simulink model "LAB1_Model1DOF_Controller"  (R2021a)
settings: Solver=VariableStepAuto  StartTime=0.0  StopTime=5  RelTol=1e-3
libraries: fl_lib x9, nesl_utility x6, dspfdesign x2, pid_lib x2, ee_lib x1, simulink x1
settings Model: Creator=matas  LastModifiedBy=10907
settings SolverCC: AlgebraicLoopSolver=TrustRegion
settings DebuggingCC: SFMachineParentedDataDiag=warning

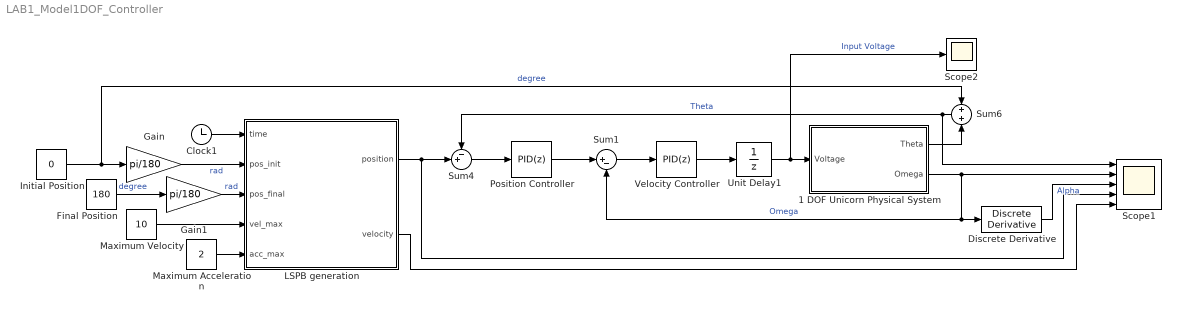
== system LAB1_Model1DOF_Controller ==
  1 DOF Unicorn Physical System : Subsystem  mask{I=0.1, b=0.01}
      mask prompts: I "Inertia"; b "Damping"
  Clock1 : Clock
  Discrete Derivative : simulink/Discrete/Discrete Derivative  gainval=1.0  ICPrevScaledInput=0.0  OutMin=[]  OutMax=[]  OutDataType=fixdt(1, 16)  OutScaling=2^-10  DoSatur=off
  Final Position : Constant  Value=180
  Gain : Gain  Gain=pi/180
  Gain1 : Gain  Gain=pi/180
  Initial Position : Constant  Value=0
  LSPB generation : MATLAB Function  TreatAsAtomicUnit=on
  Maximum Acceleration : Constant  Value=2
  Maximum Velocity : Constant  Value=10
  Position Controller : pid_lib/PID Controller  Controller=PID  Form=Parallel  TimeDomain=Discrete-time  UseExternalTs=off  SampleTime=1e-3  IntegratorMethod=Forward Euler  FilterMethod=Forward Euler  ControllerParametersSource=internal  P=150  I=100  D=10  UseFilter=on  N=100  TunerSelectOption=Transfer Function Based (PID Tuner App)  InitialConditionSource=internal  InitialConditionForIntegrator=0  InitialConditionForFilter=0  DifferentiatorICPrevScaledInput=0  ExternalReset=none  TrackingMode=off  Kt=1  LimitOutput=off  SatLimitsSource=internal  UpperSaturationLimit=2  LowerSaturationLimit=0  LinearizeAsGain=off  AntiWindupMode=none  Kb=1  POutMin=[]  POutMax=[]  IOutMin=[]  IOutMax=[]  DOutMin=[]  DOutMax=[]  NOutMin=[]  NOutMax=[]  SumOutMin=[]  SumOutMax=[]  SaturationOutMin=[]  SaturationOutMax=[]  PParamMin=[]  PParamMax=[]  IParamMin=[]  IParamMax=[]  DParamMin=[]  DParamMax=[]  NParamMin=[]  NParamMax=[]  KbParamMin=[]  KbParamMax=[]  KtParamMin=[]  KtParamMax=[]  KbOutMin=[]  KbOutMax=[]  KtOutMin=[]  KtOutMax=[]  IntegratorOutMin=[]  IntegratorOutMax=[]  FilterOutMin=[]  FilterOutMax=[]  SumI1OutMin=[]  SumI1OutMax=[]  SumI2OutMin=[]  SumI2OutMax=[]  SumI3OutMin=[]  SumI3OutMax=[]  SumI4OutMin=[]  SumI4OutMax=[]  SumDOutMin=[]  SumDOutMax=[]  DifferentiatorOutMin=[]  DifferentiatorOutMax=[]  FilterDiffOutCoefMin=[]  FilterDiffOutCoefMax=[]  ReciprocalOutMin=[]  ReciprocalOutMax=[]  SumDenOutMin=[]  SumDenOutMax=[]  SumNumOutMin=[]  SumNumOutMax=[]  DivideOutMin=[]  DivideOutMax=[]  UdiffTsProdOutMin=[]  UdiffTsProdOutMax=[]  NTsProdOutMin=[]  NTsProdOutMax=[]  UintegralTsProdOutMin=[]  UintegralTsProdOutMax=[]  UngainTsProdOutMin=[]  UngainTsProdOutMax=[]  IntegratorContinuousStateAttributes=''  IntegratorStateMustResolveToSignalObject=off  IntegratorRTWStateStorageClass=Auto  FilterContinuousStateAttributes=''  FilterStateMustResolveToSignalObject=off  FilterRTWStateStorageClass=Auto  ParallelPVariant=InternalParameters  IdealPVariant=Disabled  IVariant=InternalParameters  DVariant=InternalParameters  IntegratorVariant=Discrete  SatVariant=Disabled  AWVariant=Passthrough  PCopyVariant=Disabled  TRVariant=Disabled  FdbkBlocksVariant=Forward  IdealPFdbkVariant=Disabled  SatFdbkVariant=Disabled  DerivativeFilterVariant=ForwardEulerFilter  NVariant=InternalParameters  NCopyVariant=Disabled  FilterICVariant=InternalICsFilter  IntegratorICVariant=InternalICs  ExternalResetVariant=Disabled  TRSumVariant=Passthrough  SumFdbkVariant=Disabled  SumVariant=Sum_PID  TsampFilterVariant=InternalTs  TsampNgainVariant=Passthrough  TsampIntegralVariant=Passthrough  ExternalSaturationOutDataTypeStr=Inherit: Same as second input
  Scope1 : Scope  NumInputPorts=5
  Scope2 : Scope
  Sum1 : Sum  Inputs=|+-
  Sum4 : Sum  Inputs=-+|
  Sum6 : Sum  Inputs=+|+
  Unit Delay1 : UnitDelay  SampleTime=1/1000  HasFrameUpgradeWarning=on
  Velocity Controller : pid_lib/PID Controller  Controller=PID  Form=Parallel  TimeDomain=Discrete-time  UseExternalTs=off  SampleTime=1e-3  IntegratorMethod=Forward Euler  FilterMethod=Forward Euler  ControllerParametersSource=internal  P=0.05  I=0.5  D=0  UseFilter=on  N=100  TunerSelectOption=Transfer Function Based (PID Tuner App)  InitialConditionSource=internal  InitialConditionForIntegrator=0  InitialConditionForFilter=0  DifferentiatorICPrevScaledInput=0  ExternalReset=none  TrackingMode=off  Kt=1  LimitOutput=off  SatLimitsSource=internal  UpperSaturationLimit=2  LowerSaturationLimit=0  LinearizeAsGain=off  AntiWindupMode=none  Kb=1  POutMin=[]  POutMax=[]  IOutMin=[]  IOutMax=[]  DOutMin=[]  DOutMax=[]  NOutMin=[]  NOutMax=[]  SumOutMin=[]  SumOutMax=[]  SaturationOutMin=[]  SaturationOutMax=[]  PParamMin=[]  PParamMax=[]  IParamMin=[]  IParamMax=[]  DParamMin=[]  DParamMax=[]  NParamMin=[]  NParamMax=[]  KbParamMin=[]  KbParamMax=[]  KtParamMin=[]  KtParamMax=[]  KbOutMin=[]  KbOutMax=[]  KtOutMin=[]  KtOutMax=[]  IntegratorOutMin=[]  IntegratorOutMax=[]  FilterOutMin=[]  FilterOutMax=[]  SumI1OutMin=[]  SumI1OutMax=[]  SumI2OutMin=[]  SumI2OutMax=[]  SumI3OutMin=[]  SumI3OutMax=[]  SumI4OutMin=[]  SumI4OutMax=[]  SumDOutMin=[]  SumDOutMax=[]  DifferentiatorOutMin=[]  DifferentiatorOutMax=[]  FilterDiffOutCoefMin=[]  FilterDiffOutCoefMax=[]  ReciprocalOutMin=[]  ReciprocalOutMax=[]  SumDenOutMin=[]  SumDenOutMax=[]  SumNumOutMin=[]  SumNumOutMax=[]  DivideOutMin=[]  DivideOutMax=[]  UdiffTsProdOutMin=[]  UdiffTsProdOutMax=[]  NTsProdOutMin=[]  NTsProdOutMax=[]  UintegralTsProdOutMin=[]  UintegralTsProdOutMax=[]  UngainTsProdOutMin=[]  UngainTsProdOutMax=[]  IntegratorContinuousStateAttributes=''  IntegratorStateMustResolveToSignalObject=off  IntegratorRTWStateStorageClass=Auto  FilterContinuousStateAttributes=''  FilterStateMustResolveToSignalObject=off  FilterRTWStateStorageClass=Auto  ParallelPVariant=InternalParameters  IdealPVariant=Disabled  IVariant=InternalParameters  DVariant=InternalParameters  IntegratorVariant=Discrete  SatVariant=Disabled  AWVariant=Passthrough  PCopyVariant=Disabled  TRVariant=Disabled  FdbkBlocksVariant=Forward  IdealPFdbkVariant=Disabled  SatFdbkVariant=Disabled  DerivativeFilterVariant=ForwardEulerFilter  NVariant=InternalParameters  NCopyVariant=Disabled  FilterICVariant=InternalICsFilter  IntegratorICVariant=InternalICs  ExternalResetVariant=Disabled  TRSumVariant=Passthrough  SumFdbkVariant=Disabled  SumVariant=Sum_PID  TsampFilterVariant=InternalTs  TsampNgainVariant=Passthrough  TsampIntegralVariant=Passthrough  ExternalSaturationOutDataTypeStr=Inherit: Same as second input
  wires:
  Final Position/1 -> Gain1/1  "degree"
  Initial Position/1 -> Sum6/1, Gain/1  "degree"
  Maximum Acceleration/1 -> LSPB generation/5(acc_max)
  Maximum Velocity/1 -> LSPB generation/4(vel_max)
  Clock1/1 -> LSPB generation/1(time)
  LSPB generation/2(velocity) -> Scope1/5
  LSPB generation/1(position) -> Sum4/2, Scope1/4
  Velocity Controller/1 -> Unit Delay1/1
  1 DOF Unicorn Physical System/2(Omega) -> Discrete Derivative/1, Sum1/2, Scope1/2  "Omega"
  1 DOF Unicorn Physical System/1(Theta) -> Sum6/2
  Sum1/1 -> Velocity Controller/1
  Sum4/1 -> Position Controller/1
  Position Controller/1 -> Sum1/1
  Unit Delay1/1 -> Scope2/1, 1 DOF Unicorn Physical System/1(Voltage)  "Input Voltage"
  Discrete Derivative/1 -> Scope1/3  "Alpha"
  Sum6/1 -> Scope1/1, Sum4/1  "Theta"
  Gain/1 -> LSPB generation/2(pos_init)  "rad"
  Gain1/1 -> LSPB generation/3(pos_final)  "rad"

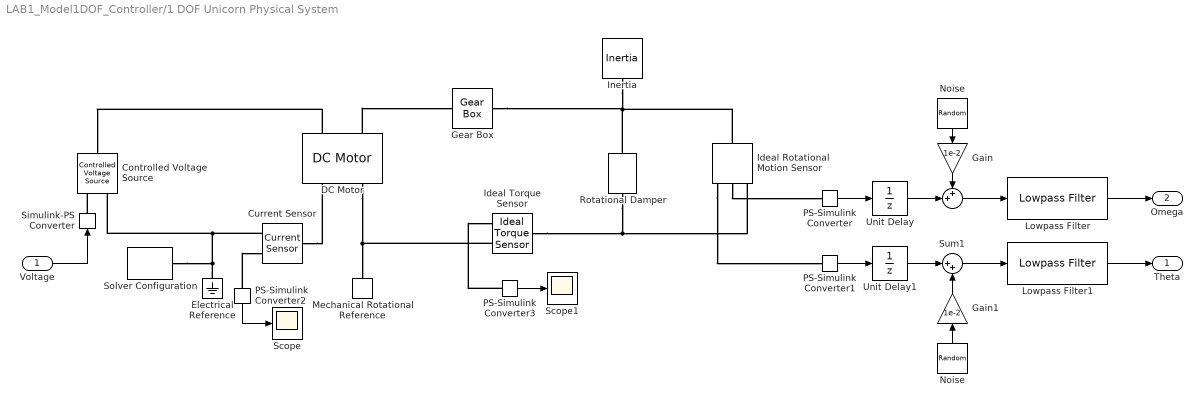
== system LAB1_Model1DOF_Controller/1 DOF Unicorn Physical System ==
  Voltage : Inport
  " " : Sum  Inputs=++|
  Controlled Voltage Source : fl_lib/Electrical/Electrical Sources/Controlled Voltage Source
  Current Sensor : fl_lib/Electrical/Electrical Sensors/Current Sensor
  "DC Motor " : ee_lib/Electromechanical/Brushed Motors/DC Motor  field_option=ee.enum.field_option.pm  Rf=100 Ohm  Lf=1 H  Laf=0.15 H  If0=0 A  parameterization=ee.enum.dcparam_option.load_speed  Ra=3.9 Ohm  La=65 uH  emf_or_torque=ee.enum.emf_or_torque.kv  Kv=0.072e-3 V/rpm  Ki=6.876e-4 N*m/A  T_stall=0.24e-3 N*m  w_max=8100 rpm  w_rated=7700 rpm  P_rated=17 W  V_rated=12 V  J=0.01 g*cm^2  lam_param=ee.enum.lam_param.current  lam=0 N*m/(rad/s)  i_noload=0.075 A  V_i_noload=12 V  speed0=0 rpm  enable_fault_armature=ee.enum.faults.faultEnable.no  rev_faulted=1 / 3  G_faulted_armature=1e-5 S  fault_trigger_armature=ee.enum.faults.faultTrigger.temporal  t_fault_armature=1 s  max_permissible_current_armature=inf A  t_fail_on_current_armature=1 s  enable_fault_field=ee.enum.faults.faultEnable.no  G_faulted_field=1e-5 S  fault_trigger_field=ee.enum.faults.faultTrigger.temporal  t_fault_field=1 s  max_permissible_current_field=inf A  t_fail_on_current_field=1 s  fault_action=ee.enum.faults.faultAction.none  alpha=3.93e-3 1/K  Tmeas=25 degC  thermal_mass=100 J/K  initial_temperature=25 degC
  Electrical Reference : fl_lib/Electrical/Electrical Elements/Electrical Reference
  Gain : Gain  Gain=1e-2
  Gain1 : Gain  Gain=1e-2
  Gear Box : fl_lib/Mechanical/Mechanisms/Gear Box  ratio=64  t_in_specify=off  t_in_priority=None  t_in=0 N*m  t_in_nominal_specify=off  t_in_nominal_unit=N*m  t_in_nominal_value=1  t_out_specify=off  t_out_priority=None  t_out=0 N*m  t_out_nominal_specify=off  t_out_nominal_unit=N*m  t_out_nominal_value=1
  Ideal Rotational Motion Sensor : fl_lib/Mechanical/Mechanical Sensors/Ideal Rotational Motion Sensor  wrap_angle=simscape.enum.onoff.off  offset=0 rad
  Ideal Torque Sensor : fl_lib/Mechanical/Mechanical Sensors/Ideal Torque Sensor
  Inertia : fl_lib/Mechanical/Rotational Elements/Inertia  inertia=I kg*m^2  num_ports=foundation.enum.numPorts2.one  w_specify=off  w_priority=High  w=0 rad/s  w_nominal_specify=off  w_nominal_unit=rad/s  w_nominal_value=1  t_specify=off  t_priority=None  t=0 N*m  t_nominal_specify=off  t_nominal_unit=N*m  t_nominal_value=1
  Lowpass Filter : dspfdesign/Lowpass Filter  FilterType=FIR  DesignForMinimumOrder=on  FilterOrder=50  PassbandFrequency=1.6  StopbandFrequency=30  PassbandRipple=0.1  StopbandAttenuation=40  InheritSampleRate=on  SampleRate=44100  SimulateUsing=Interpreted execution  roundingMode=Floor  coeffsDataTypeStr=fixdt(1,16)
  Lowpass Filter1 : dspfdesign/Lowpass Filter  FilterType=FIR  DesignForMinimumOrder=on  FilterOrder=50  PassbandFrequency=1.6  StopbandFrequency=30  PassbandRipple=0.1  StopbandAttenuation=40  InheritSampleRate=on  SampleRate=44100  SimulateUsing=Interpreted execution  roundingMode=Floor  coeffsDataTypeStr=fixdt(1,16)
  Mechanical Rotational Reference : fl_lib/Mechanical/Rotational Elements/Mechanical Rotational Reference
  Noise : RandomNumber  Variance=1/100000  SampleTime=1/1000
  "Noise " : RandomNumber  Variance=1/100000  SampleTime=1/100
  PS-Simulink Converter{,1..3} (4 alike) : nesl_utility/PS-Simulink Converter  PhysicalDomain=network_engine_domain  SubClassName=ps_output  LeftPortType=input  RightPortType=output  PseudoPeriodic=off  Frequencies=[]  Unit=inherit  AffineConversion=off
      settings: SourceProductBaseCode=PW,SS
  Rotational Damper : fl_lib/Mechanical/Rotational Elements/Rotational Damper  D=b N*m/(rad/s)  w_specify=off  w_priority=None  w=0 rad/s  w_nominal_specify=off  w_nominal_unit=rad/s  w_nominal_value=1  t_specify=off  t_priority=None  t=0 N*m  t_nominal_specify=off  t_nominal_unit=N*m  t_nominal_value=1
  Scope : Scope
  Scope1 : Scope
  Simulink-PS Converter : nesl_utility/Simulink-PS Converter  PhysicalDomain=network_engine_domain  SubClassName=ps_input  LeftPortType=input  RightPortType=output  PseudoPeriodic=off  Frequencies=[]  NoiseDistribution=none  NoiseParameters=[]  Unit=1  AffineConversion=off  FilteringAndDerivatives=provide  SimscapeFilterOrder=1  InputFilterTimeConstant=0.001  UdotUserProvided=0
      settings: SourceProductBaseCode=PW,SS
  Solver Configuration : nesl_utility/Solver Configuration  PhysicalDomain=network_engine_domain  SubClassName=solver  LeftPortType=input  RightPortType=generic  Tones=[]  Harmonics=[]  SimulateNoise=off  Profile=off  UseLocalSampling=off  EnableSwitchedLinearOptims=on  FrequencyDomain=off  UseCCode=off  RelTol=0.001  AbsTol=1e-06  MinStep=1e-09  ToWorkspace=off  RevertToSquareIcSolve=off  NumHomotopyIterations=100  PhasorMode=off  PhasorModeNumHarmonics=1  DoDC=off  ResidualTolerance=1e-09  UseLocalSolver=off  LocalSolverChoice=NE_BACKWARD_EULER_ADVANCER  LocalSolverSampleTime=0.001  DoFixedCost=off  MaxNonlinIter=3  MaxModeIter=2  ComputeImpulses=off  ImpulseIterations=2  LinearAlgebra=auto  EquationFormulation=NE_TIME_EF  DelaysMemoryBudget=1024  AutomaticFiltering=on  FilteringTimeConstant=0.001  PartitionStorageMethod=AS_NEEDED  PartitionMemoryBudget=1024  PartitionMethod=ROBUST
      settings: SourceProductBaseCode=PW,SS
  Sum1 : Sum  Inputs=|++
  Unit Delay : UnitDelay  SampleTime=1/1000  HasFrameUpgradeWarning=on
  Unit Delay1 : UnitDelay  SampleTime=1/1000  HasFrameUpgradeWarning=on
  Theta : Outport
  Omega : Outport  Port=2
  wires:
  PS-Simulink Converter/1 -> Unit Delay/1
  PS-Simulink Converter2/1 -> Scope/1
  PS-Simulink Converter3/1 -> Scope1/1
  Noise/1 -> Gain/1
  Unit Delay/1 -> " "/2
  Lowpass Filter/1 -> Omega/1
  "Noise "/1 -> Gain1/1
  Unit Delay1/1 -> Sum1/1
  Sum1/1 -> Lowpass Filter1/1
  PS-Simulink Converter1/1 -> Unit Delay1/1
  Lowpass Filter1/1 -> Theta/1
  Voltage/1 -> Simulink-PS Converter/1
  " "/1 -> Lowpass Filter/1
  Gain1/1 -> Sum1/2
  Gain/1 -> " "/1
  connections:
  Solver Configuration/RConn1 -- Electrical Reference/LConn1 -- Current Sensor/RConn2 -- Controlled Voltage Source/RConn2
  Rotational Damper/LConn1 -- Gear Box/RConn1 -- Inertia/LConn1 -- Ideal Rotational Motion Sensor/LConn1
  Simulink-PS Converter/RConn1 -- Controlled Voltage Source/RConn1
  Ideal Rotational Motion Sensor/RConn3 -- PS-Simulink Converter1/LConn1
  Ideal Rotational Motion Sensor/RConn2 -- PS-Simulink Converter/LConn1
  PS-Simulink Converter2/LConn1 -- Current Sensor/RConn1
  Rotational Damper/RConn1 -- Ideal Torque Sensor/LConn1 -- Ideal Rotational Motion Sensor/RConn1
  Ideal Torque Sensor/RConn1 -- "DC Motor "/RConn2 -- Mechanical Rotational Reference/LConn1
  PS-Simulink Converter3/LConn1 -- Ideal Torque Sensor/RConn2
  Current Sensor/LConn1 -- "DC Motor "/RConn1
  "DC Motor "/LConn2 -- Gear Box/LConn1
  "DC Motor "/LConn1 -- Controlled Voltage Source/LConn1

== matlab function LAB1_Model1DOF_Controller/LSPB generation ==
  data: time input; position output; pos_init input; pos_final input; vel_max input; acc_max input; velocity output
function [position, velocity] = fcn(time, pos_init, pos_final, vel_max, acc_max)
s = (pos_final-pos_init);

if (abs(vel_max)^2)/2/abs(acc_max) >= abs(s)/2 
    Tb = sqrt(abs(s)/acc_max);
    
    if time < Tb
        position = 0.5*acc_max*(time^2) + pos_init;
        velocity = acc_max*time;
    elseif time < 2*Tb
        position = sqrt(acc_max*abs(s))*(time-Tb) - 0.5*acc_max*((time-Tb)^2) + abs(s)/2 + pos_init;
        velocity = sqrt(acc_max*abs(s)) - acc_max*(time-Tb);
    else
        position = pos_init + abs(s);
        velocity = 0;
    end
    
else
    Tb = vel_max/acc_max;
    Ts = (abs(s) - (vel_max^2)/acc_max) /vel_max;
    
    if time < Tb
        position = 0.5*acc_max*(time^2) + pos_init;
        velocity = acc_max*time;
    elseif time < Tb+Ts
        position = vel_max*(time-Tb) + (vel_max^2)/2/acc_max + pos_init;
        velocity = vel_max;
    elseif time < Tb+Ts+Tb
        position = vel_max*(time-Tb-Ts) - 0.5*acc_max*((time-Tb-Ts)^2) + (s - (vel_max^2)/2/acc_max) + pos_init;
        velocity = vel_max - acc_max*(time-Tb-Ts);
    else
        position = pos_init + abs(s);
        velocity = 0;
    end
end

if (pos_init>pi)||(pos_init<-pi)||(pos_final>pi)||(pos_final<-pi)
    position = 0;
    velocity = 0;
elseif s < 0
    position = -position;
    velocity = -velocity;
end
